simulink model "CTRL_ADAPT"  (R2023a)
settings: Solver=ode1  StartTime=0.0  StopTime=25  FixedStep=Ts  RelTol=1e-3
values from neighbouring files (symbols this model uses):
  Ts = 0.001    [TRAJ.m]
undefined symbols (not defined in the file or in its folder): DiscIntNeverNeededParam, PI0
settings Model: Creator=39388  LastModifiedBy=39388

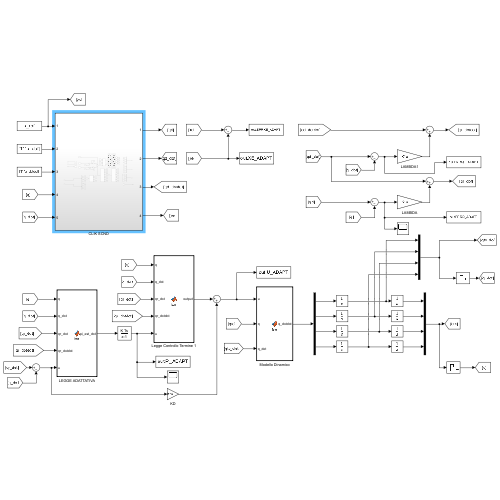
[thumbnail: Simulink's stored preview of the top-level diagram]
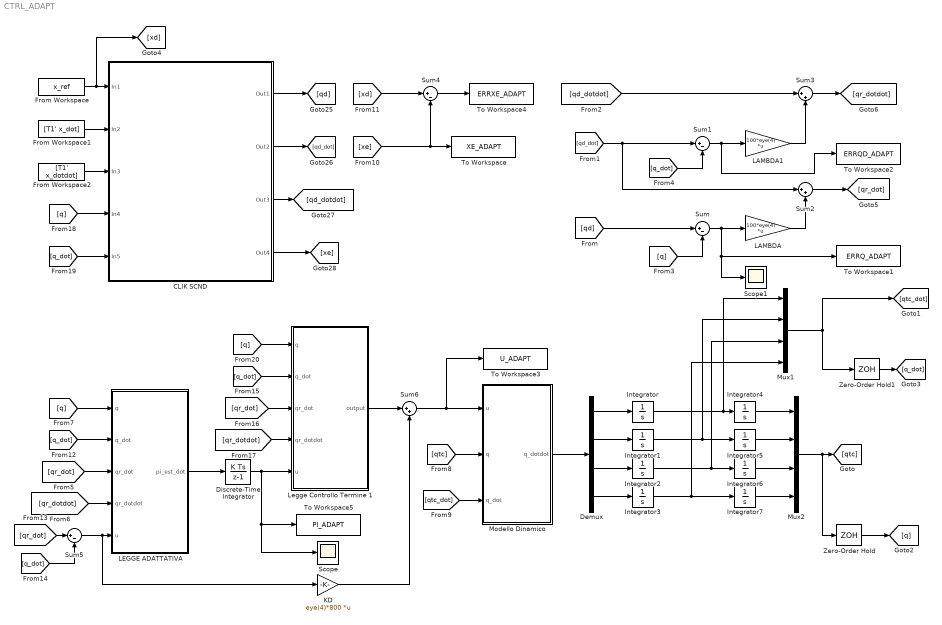
== system CTRL_ADAPT ==
  CLIK SCND : Subsystem
  Demux : Demux
  Discrete-Time Integrator : DiscreteIntegrator  InitialCondition=PI0'  SampleTime=Ts  ICPrevOutput=DiscIntNeverNeededParam  ICPrevScaledInput=DiscIntNeverNeededParam
  From Workspace : FromWorkspace  VariableName=x_ref  SampleTime=Ts
  From Workspace1 : FromWorkspace  VariableName=[T1' x_dot]  SampleTime=Ts
  From Workspace2 : FromWorkspace  VariableName=[T1' x_dotdot]  SampleTime=Ts
  Integrator : Integrator  UpperSaturationLimit=50  LowerSaturationLimit=-50
  Integrator{1..4} (4 alike) : Integrator
  Integrator5 : Integrator  InitialCondition=pi/2
  Integrator6 : Integrator  InitialCondition=-0.25
  Integrator7 : Integrator  InitialCondition=-pi
  KD : Gain  Gain=eye(4)*800  Multiplication=Matrix(K*u)
  LAMBDA : Gain  Gain=100*eye(4)  Multiplication=Matrix(K*u)
  LAMBDA1 : Gain  Gain=100*eye(4)  Multiplication=Matrix(K*u)
  LEGGE ADATTATIVA : MATLAB Function  TreatAsAtomicUnit=on
  Legge Controllo Termine 1 : MATLAB Function  TreatAsAtomicUnit=on
  Modello Dinamico : MATLAB Function  TreatAsAtomicUnit=on
  Mux1 : Mux
  Mux2 : Mux
  Scope : Scope
  Scope1 : Scope
  Sum{,1,4..5} (4 alike) : Sum  Inputs=|+-
  Sum2 : Sum  Inputs=|++
  Sum3 : Sum  Inputs=|++
  Sum6 : Sum  Inputs=|++
  To Workspace : ToWorkspace  VariableName=XE_ADAPT  SaveFormat=Structure With Time  SampleTime=-1
  To Workspace1 : ToWorkspace  VariableName=ERRQ_ADAPT  SaveFormat=Structure With Time  SampleTime=-1
  To Workspace2 : ToWorkspace  VariableName=ERRQD_ADAPT  SaveFormat=Structure With Time  SampleTime=-1
  To Workspace3 : ToWorkspace  VariableName=U_ADAPT  SaveFormat=Structure With Time  SampleTime=-1
  To Workspace4 : ToWorkspace  VariableName=ERRXE_ADAPT  SaveFormat=Structure With Time  SampleTime=-1
  To Workspace5 : ToWorkspace  VariableName=PI_ADAPT  SaveFormat=Structure With Time  SampleTime=-1
  Zero-Order Hold : ZeroOrderHold  SampleTime=Ts
  Zero-Order Hold1 : ZeroOrderHold  SampleTime=Ts
  wires:
  From Workspace/1 -> [xd], CLIK SCND/1(In1)
  From Workspace1/1 -> CLIK SCND/2(In2)
  From Workspace2/1 -> CLIK SCND/3(In3)
  [q] -> CLIK SCND/4(In4)
  [q_dot] -> CLIK SCND/5(In5)
  CLIK SCND/1(Out1) -> [qd]
  CLIK SCND/2(Out2) -> [qd_dot]
  CLIK SCND/3(Out3) -> [qd_dotdot]
  CLIK SCND/4(Out4) -> [xe]
  [qtc] -> Modello Dinamico/2(q)
  [qtc_dot] -> Modello Dinamico/3(q_dot)
  Modello Dinamico/1(q_dotdot) -> Demux/1
  Demux/1 -> Integrator/1
  Demux/2 -> Integrator1/1
  Demux/3 -> Integrator2/1
  Demux/4 -> Integrator3/1
  Integrator/1 -> Mux1/1, Integrator4/1
  Integrator1/1 -> Mux1/2, Integrator5/1
  Integrator2/1 -> Mux1/3, Integrator6/1
  Integrator3/1 -> Mux1/4, Integrator7/1
  Integrator4/1 -> Mux2/1
  Integrator5/1 -> Mux2/2
  Integrator6/1 -> Mux2/3
  Integrator7/1 -> Mux2/4
  Mux2/1 -> Zero-Order Hold/1, [qtc]
  Mux1/1 -> Zero-Order Hold1/1, [qtc_dot]
  Zero-Order Hold/1 -> [q]
  Zero-Order Hold1/1 -> [q_dot]
  [xe] -> Sum4/2, To Workspace/1
  [xd] -> Sum4/1
  Sum4/1 -> To Workspace4/1
  [qd_dot] -> Sum2/1, Sum1/1
  [q_dot] -> Sum1/2
  [qd] -> Sum/1
  [q] -> Sum/2
  Sum/1 -> Scope1/1, To Workspace1/1, LAMBDA/1
  LAMBDA/1 -> Sum2/2
  Sum2/1 -> [qr_dot]
  [qr_dot] -> LEGGE ADATTATIVA/3(qr_dot)
  Sum1/1 -> To Workspace2/1, LAMBDA1/1
  LAMBDA1/1 -> Sum3/2
  [qd_dotdot] -> Sum3/1
  Sum3/1 -> [qr_dotdot]
  [qr_dotdot] -> LEGGE ADATTATIVA/4(qr_dotdot)
  [q] -> LEGGE ADATTATIVA/1(q)
  [q_dot] -> LEGGE ADATTATIVA/2(q_dot)
  [q_dot] -> Sum5/2
  Sum5/1 -> KD/1, LEGGE ADATTATIVA/5(u)
  [qr_dot] -> Sum5/1
  LEGGE ADATTATIVA/1(pi_est_dot) -> Discrete-Time Integrator/1
  Discrete-Time Integrator/1 -> Scope/1, To Workspace5/1, Legge Controllo Termine 1/5(u)
  [q_dot] -> Legge Controllo Termine 1/2(q_dot)
  [qr_dot] -> Legge Controllo Termine 1/3(qr_dot)
  [q] -> Legge Controllo Termine 1/1(q)
  [qr_dotdot] -> Legge Controllo Termine 1/4(qr_dotdot)
  Sum6/1 -> To Workspace3/1, Modello Dinamico/1(u)
  Legge Controllo Termine 1/1(output) -> Sum6/1
  KD/1 -> Sum6/2

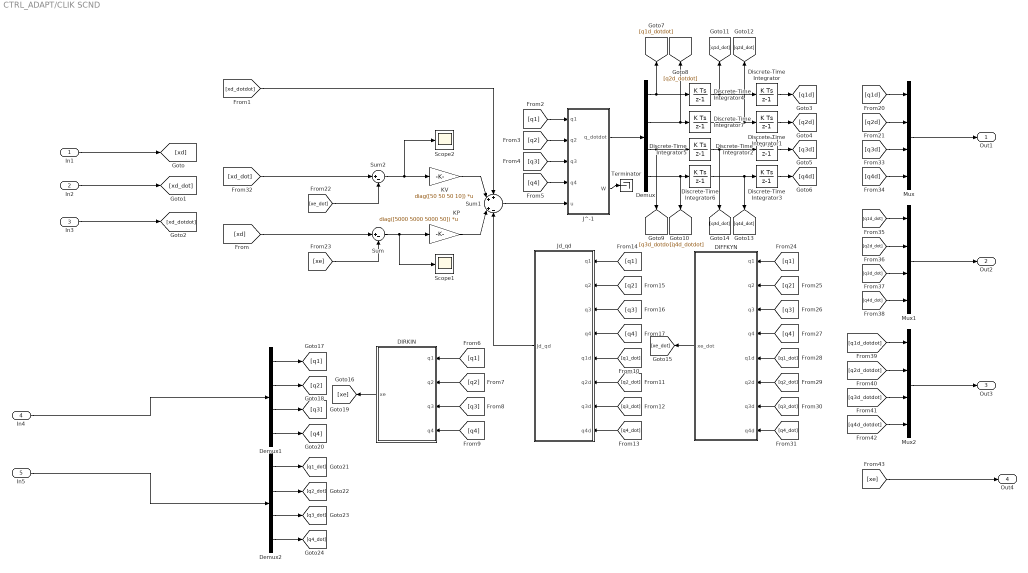
== system CTRL_ADAPT/CLIK SCND ==
  In1 : Inport
  In2 : Inport  Port=2
  In3 : Inport  Port=3
  In4 : Inport  Port=4
  In5 : Inport  Port=5
  DIFFKYN : MATLAB Function  TreatAsAtomicUnit=on
  DIRKIN : MATLAB Function  TreatAsAtomicUnit=on
  Demux : Demux
  Demux1 : Demux
  Demux2 : Demux
  Discrete-Time Integrator{,4..7} (5 alike) : DiscreteIntegrator  SampleTime=Ts  ICPrevOutput=DiscIntNeverNeededParam  ICPrevScaledInput=DiscIntNeverNeededParam
  Discrete-Time Integrator1 : DiscreteIntegrator  InitialCondition=pi/2  SampleTime=Ts  ICPrevOutput=DiscIntNeverNeededParam  ICPrevScaledInput=DiscIntNeverNeededParam
  Discrete-Time Integrator2 : DiscreteIntegrator  InitialCondition=-0.25  SampleTime=Ts  ICPrevOutput=DiscIntNeverNeededParam  ICPrevScaledInput=DiscIntNeverNeededParam
  Discrete-Time Integrator3 : DiscreteIntegrator  InitialCondition=-pi  SampleTime=Ts  ICPrevOutput=DiscIntNeverNeededParam  ICPrevScaledInput=DiscIntNeverNeededParam
  J^-1 : MATLAB Function  TreatAsAtomicUnit=on
  Jd_qd : MATLAB Function  TreatAsAtomicUnit=on
  KP : Gain  Gain=diag([5000 5000 5000 50])  Multiplication=Matrix(K*u)
  KV : Gain  Gain=diag([50 50 50 10])  Multiplication=Matrix(K*u)
  Mux : Mux
  Mux1 : Mux
  Mux2 : Mux
  Scope1 : Scope
  Scope2 : Scope
  Sum : Sum  Inputs=|+-
  Sum1 : Sum  Inputs=++|+-
  Sum2 : Sum  Inputs=|+-
  Terminator : Terminator
  Out1 : Outport
  Out2 : Outport  Port=2
  Out3 : Outport  Port=3
  Out4 : Outport  Port=4
  wires:
  [q4] -> J^-1/4(q4)
  [q1] -> DIFFKYN/1(q1)
  Demux/3 -> [q3d_dotdot], Discrete-Time Integrator5/1
  [q2d] -> Mux/2
  Discrete-Time Integrator1/1 -> [q2d]
  In5/1 -> Demux2/1
  [q1] -> DIRKIN/1(q1)
  [q4] -> DIRKIN/4(q4)
  Discrete-Time Integrator/1 -> [q1d]
  Demux/1 -> Discrete-Time Integrator4/1, [q1d_dotdot]
  Discrete-Time Integrator5/1 -> [q3d_dot], Discrete-Time Integrator2/1
  [xe_dot] -> Sum2/2
  [q3] -> J^-1/3(q3)
  [q3d] -> Mux/3
  Demux/4 -> [q4d_dotdot], Discrete-Time Integrator6/1
  [q1_dot] -> DIFFKYN/5(q1d)
  [q2] -> J^-1/2(q2)
  [q3] -> DIRKIN/3(q3)
  In2/1 -> [xd_dot]
  J^-1/1(q_dotdot) -> Demux/1
  Discrete-Time Integrator2/1 -> [q3d]
  [q2_dot] -> DIFFKYN/6(q2d)
  [xd] -> Sum/1
  Sum1/1 -> J^-1/5(u)
  [q4d] -> Mux/4
  KV/1 -> Sum1/2
  Jd_qd/1(Jd_qd) -> Sum1/4
  Discrete-Time Integrator3/1 -> [q4d]
  Discrete-Time Integrator4/1 -> [q1d_dot], Discrete-Time Integrator/1
  [q4d_dot] -> Mux1/4
  Demux1/3 -> [q3]
  Discrete-Time Integrator7/1 -> [q2d_dot], Discrete-Time Integrator1/1
  [xd_dotdot] -> Sum1/1
  [q2d_dot] -> Mux1/2
  Sum/1 -> Scope1/1, KP/1
  [xe] -> Sum/2
  Discrete-Time Integrator6/1 -> [q4d_dot], Discrete-Time Integrator3/1
  [q1] -> Jd_qd/1(q1)
  [q3_dot] -> DIFFKYN/7(q3d)
  [q2] -> DIFFKYN/2(q2)
  KP/1 -> Sum1/3
  [q3] -> Jd_qd/3(q3)
  In3/1 -> [xd_dotdot]
  [q3d_dot] -> Mux1/3
  DIRKIN/1(xe) -> [xe]
  [q3] -> DIFFKYN/3(q3)
  Demux1/2 -> [q2]
  [q1] -> J^-1/1(q1)
  [q2] -> Jd_qd/2(q2)
  Demux/2 -> [q2d_dotdot], Discrete-Time Integrator7/1
  [xe] -> Out4/1
  [q2] -> DIRKIN/2(q2)
  [q4_dot] -> DIFFKYN/8(q4d)
  [q4] -> Jd_qd/4(q4)
  DIFFKYN/1(xe_dot) -> [xe_dot]
  [xd_dot] -> Sum2/1
  J^-1/2(W) -> Terminator/1
  [q4] -> DIFFKYN/4(q4)
  Demux2/3 -> [q3_dot]
  Sum2/1 -> Scope2/1, KV/1
  [q3d_dotdot] -> Mux2/3
  [q1d_dot] -> Mux1/1
  [q1d] -> Mux/1
  Demux2/4 -> [q4_dot]
  Demux2/1 -> [q1_dot]
  Demux2/2 -> [q2_dot]
  [q4_dot] -> Jd_qd/8(q4d)
  [q1_dot] -> Jd_qd/5(q1d)
  [q3_dot] -> Jd_qd/7(q3d)
  [q2_dot] -> Jd_qd/6(q2d)
  [q1d_dotdot] -> Mux2/1
  [q4d_dotdot] -> Mux2/4
  [q2d_dotdot] -> Mux2/2
  Demux1/1 -> [q1]
  Demux1/4 -> [q4]
  In4/1 -> Demux1/1
  In1/1 -> [xd]
  Mux1/1 -> Out2/1
  Mux/1 -> Out1/1
  Mux2/1 -> Out3/1

== matlab function CTRL_ADAPT/CLIK SCND/DIRKIN ==
  data: q1 input; xe output; q2 input; q3 input; q4 input
function xe = fcn(q1,q2,q3,q4)

xe=[0.5*cos(q1)+0.5*cos(q1+q2);
    0.5*sin(q1)+0.5*sin(q1+q2);
    1+q3;
    q1+q2+q4];

== matlab function CTRL_ADAPT/CLIK SCND/J^-1 ==
  data: q1 input; q2 input; q3 input; q4 input; u input; q_dotdot output; W output
function  [q_dotdot,W] = fcn(q1,q2,q3,q4,u)

    J=[-0.5*sin(q1-0.5*sin(q1+q2)) -0.5*sin(q1+q2) 0 0;
        0.5*cos(q1-0.5*cos(q1+q2))  0.5*cos(q1+q2) 0 0;
        0                               0                 1 0;
        1                               1                 0 1];

     q_dotdot=J\u;
     
     W=0.5^2*abs(sin(q2));

== matlab function CTRL_ADAPT/CLIK SCND/Jd_qd ==
  data: q1 input; Jd_qd output; q2 input; q3 input; q4 input; q1d input; q2d input; q3d input; q4d input
function Jd_qd = fcn(q1,q2,q3,q4,q1d,q2d,q3d,q4d)

J_dot=[-0.5*q1d*cos(q1)-0.5*(q1d+q2d)*cos(q1+q2) -0.5*(q1d+q2d)*cos(q1+q2) 0 0;
       -0.5*q1d*sin(q1)-0.5*(q1d+q2d)*sin(q1+q2) -0.5*(q1d+q2d)*sin(q1+q2) 0 0;
        0                                         0                        0 0;
        0                                         0                        0 0];

Jd_qd=J_dot*[q1d; q2d; q3d; q4d];

== matlab function CTRL_ADAPT/CLIK SCND/DIFFKYN ==
  data: q1 input; xe_dot output; q2 input; q3 input; q4 input; q1d input; q2d input; q3d input; q4d input
function xe_dot = fcn(q1,q2,q3,q4,q1d,q2d,q3d,q4d)

J=[-0.5*sin(q1-0.5*sin(q1+q2)) -0.5*sin(q1+q2) 0 0;
    0.5*cos(q1-0.5*cos(q1+q2))  0.5*cos(q1+q2) 0 0;
    0                           0              1 0;
    1                           1              0 1];

xe_dot=J*[q1d;q2d;q3d;q4d];

== matlab function CTRL_ADAPT/LEGGE ADATTATIVA ==
  data: q input; pi_est_dot output; q_dot input; qr_dot input; qr_dotdot input; u input
function pi_est_dot = fcn(q,q_dot,qr_dot,qr_dotdot,u)

Kpi=eye(17)*100;
Kpi(6,6)=0.01;

q1=q(1);
q2=q(2);
q3=q(3);
q4=q(4);
qd1=q_dot(1);
qd2=q_dot(2);
qd3=q_dot(3);
qd4=q_dot(4);
qrd1=qr_dot(1);
qrd2=qr_dot(2);
qrd3=qr_dot(3);
qrd4=qr_dot(4);
qrdd1=qr_dotdot(1);
qrdd2=qr_dotdot(2);
qrdd3=qr_dotdot(3);
qrdd4=qr_dotdot(4);

Y=[(qrdd1*(2*cos(conj(q1))*cos(q1) + 2*sin(conj(q1))*sin(q1)))/2, qrdd1*((cos(conj(q1))*cos(q1))/4 + (sin(conj(q1))*sin(q1))/4), qrdd1*((cos(conj(q1))*cos(q1 + q2))/2 + (sin(conj(q1))*sin(q1 + q2))/2 + (cos(conj(q1) + conj(q2))*cos(q1))/2 + (sin(conj(q1) + conj(q2))*sin(q1))/2) + qrdd2*((cos(conj(q1))*cos(q1 + q2))/2 + (sin(conj(q1))*sin(q1 + q2))/2) - (qd2*qrd1*sin(q2))/2 - (qrd2*sin(q2)*(qd1 + qd2))/2, (qrdd1*(2*cos(conj(q1) + conj(q2))*cos(q1 + q2) + 2*sin(conj(q1) + conj(q2))*sin(q1 + q2)))/2 + (qrdd2*(2*cos(conj(q1) + conj(q2))*cos(q1 + q2) + 2*sin(conj(q1) + conj(q2))*sin(q1 + q2)))/2, qrdd1*((cos(q1 + q2)/2 + cos(q1)/2)*(cos(conj(q1))/2 + cos(conj(q1) + conj(q2))/2) + (sin(q1 + q2)/2 + sin(q1)/2)*(sin(conj(q1))/2 + sin(conj(q1) + conj(q2))/2)) + qrdd2*((cos(q1 + q2)*(cos(conj(q1))/2 + cos(conj(q1) + conj(q2))/2))/2 + (sin(q1 + q2)*(sin(conj(q1))/2 + sin(conj(q1) + conj(q2))/2))/2) - (qd2*qrd1*sin(q2))/4 - (qrd2*sin(q2)*(qd1 + qd2))/4, qrdd1*((cos(q1 + q2)/2 + cos(q1)/2)*(cos(conj(q1))/2 + cos(conj(q1) + conj(q2))/2) + (sin(q1 + q2)/2 + sin(q1)/2)*(sin(conj(q1))/2 + sin(conj(q1) + conj(q2))/2)) + qrdd2*((cos(q1 + q2)*(cos(conj(q1))/2 + cos(conj(q1) + conj(q2))/2))/2 + (sin(q1 + q2)*(sin(conj(q1))/2 + sin(conj(q1) + conj(q2))/2))/2) - (qd2*qrd1*sin(q2))/4 - (qrd2*sin(q2)*(qd1 + qd2))/4, qrdd1, qrdd1 + qrdd2, qrdd1 + qrdd2 + qrdd4, qrdd1, qrdd1 + qrdd2,         qrdd1 + qrdd2 + 50*qrdd3,        qrdd1 + qrdd2 + 20*qrdd4, qrd1,    0,         0,        0;
                                                            0,                                                             0,                                                                                                                                                                            qrdd1*((cos(conj(q1) + conj(q2))*cos(q1))/2 + (sin(conj(q1) + conj(q2))*sin(q1))/2) + (qd1*qrd1*sin(q2))/2, (qrdd1*(2*cos(conj(q1) + conj(q2))*cos(q1 + q2) + 2*sin(conj(q1) + conj(q2))*sin(q1 + q2)))/2 + (qrdd2*(2*cos(conj(q1) + conj(q2))*cos(q1 + q2) + 2*sin(conj(q1) + conj(q2))*sin(q1 + q2)))/2,                                                                                                                qrdd1*((cos(conj(q1) + conj(q2))*(cos(q1 + q2)/2 + cos(q1)/2))/2 + (sin(conj(q1) + conj(q2))*(sin(q1 + q2)/2 + sin(q1)/2))/2) + qrdd2*((cos(conj(q1) + conj(q2))*cos(q1 + q2))/4 + (sin(conj(q1) + conj(q2))*sin(q1 + q2))/4) + (qd1*qrd1*sin(q2))/4,                                                                                                                qrdd1*((cos(conj(q1) + conj(q2))*(cos(q1 + q2)/2 + cos(q1)/2))/2 + (sin(conj(q1) + conj(q2))*(sin(q1 + q2)/2 + sin(q1)/2))/2) + qrdd2*((cos(conj(q1) + conj(q2))*cos(q1 + q2))/4 + (sin(conj(q1) + conj(q2))*sin(q1 + q2))/4) + (qd1*qrd1*sin(q2))/4,     0, qrdd1 + qrdd2, qrdd1 + qrdd2 + qrdd4,     0, qrdd1 + qrdd2,         qrdd1 + qrdd2 + 50*qrdd3,        qrdd1 + qrdd2 + 20*qrdd4,    0, qrd2,         0,        0;
                                                            0,                                                             0,                                                                                                                                                                                                                                                                                     0,                                                                                                                                                                                             0,                                                                                                                                                                                                                                                                                                                                                     qrdd3 + 981/100,                                                                                                                                                                                                                                                                                                                                                     qrdd3 + 981/100,     0,             0,                     0,     0,             0, 50*qrdd1 + 50*qrdd2 + 2500*qrdd3,                               0,    0,    0, 2500*qrd3,        0;
                                                            0,                                                             0,                                                                                                                                                                                                                                                                                     0,                                                                                                                                                                                             0,                                                                                                                                                                                                                                                                                                                                                                   0,                                                                                                                                                                                                                                                                                                                                                                   0,     0,             0, qrdd1 + qrdd2 + qrdd4,     0,             0,                                0, 20*qrdd1 + 20*qrdd2 + 400*qrdd4,    0,    0,         0, 400*qrd4];
 
pi_est_dot = inv(Kpi)*Y'*u;

== matlab function CTRL_ADAPT/Legge Controllo Termine 1 ==
  data: q input size=4; output output size=4; q_dot input size=4; qr_dot input size=4; qr_dotdot input size=4; u input size=17
function output = fcn(q,q_dot,qr_dot,qr_dotdot,u)

q1=q(1);
q2=q(2);
q3=q(3);
q4=q(4);
qd1=q_dot(1);
qd2=q_dot(2);
qd3=q_dot(3);
qd4=q_dot(4);
qrd1=qr_dot(1);
qrd2=qr_dot(2);
qrd3=qr_dot(3);
qrd4=qr_dot(4);
qrdd1=qr_dotdot(1);
qrdd2=qr_dotdot(2);
qrdd3=qr_dotdot(3);
qrdd4=qr_dotdot(4);

Y=[(qrdd1*(2*cos(conj(q1))*cos(q1) + 2*sin(conj(q1))*sin(q1)))/2, qrdd1*((cos(conj(q1))*cos(q1))/4 + (sin(conj(q1))*sin(q1))/4), qrdd1*((cos(conj(q1))*cos(q1 + q2))/2 + (sin(conj(q1))*sin(q1 + q2))/2 + (cos(conj(q1) + conj(q2))*cos(q1))/2 + (sin(conj(q1) + conj(q2))*sin(q1))/2) + qrdd2*((cos(conj(q1))*cos(q1 + q2))/2 + (sin(conj(q1))*sin(q1 + q2))/2) - (qd2*qrd1*sin(q2))/2 - (qrd2*sin(q2)*(qd1 + qd2))/2, (qrdd1*(2*cos(conj(q1) + conj(q2))*cos(q1 + q2) + 2*sin(conj(q1) + conj(q2))*sin(q1 + q2)))/2 + (qrdd2*(2*cos(conj(q1) + conj(q2))*cos(q1 + q2) + 2*sin(conj(q1) + conj(q2))*sin(q1 + q2)))/2, qrdd1*((cos(q1 + q2)/2 + cos(q1)/2)*(cos(conj(q1))/2 + cos(conj(q1) + conj(q2))/2) + (sin(q1 + q2)/2 + sin(q1)/2)*(sin(conj(q1))/2 + sin(conj(q1) + conj(q2))/2)) + qrdd2*((cos(q1 + q2)*(cos(conj(q1))/2 + cos(conj(q1) + conj(q2))/2))/2 + (sin(q1 + q2)*(sin(conj(q1))/2 + sin(conj(q1) + conj(q2))/2))/2) - (qd2*qrd1*sin(q2))/4 - (qrd2*sin(q2)*(qd1 + qd2))/4, qrdd1*((cos(q1 + q2)/2 + cos(q1)/2)*(cos(conj(q1))/2 + cos(conj(q1) + conj(q2))/2) + (sin(q1 + q2)/2 + sin(q1)/2)*(sin(conj(q1))/2 + sin(conj(q1) + conj(q2))/2)) + qrdd2*((cos(q1 + q2)*(cos(conj(q1))/2 + cos(conj(q1) + conj(q2))/2))/2 + (sin(q1 + q2)*(sin(conj(q1))/2 + sin(conj(q1) + conj(q2))/2))/2) - (qd2*qrd1*sin(q2))/4 - (qrd2*sin(q2)*(qd1 + qd2))/4, qrdd1, qrdd1 + qrdd2, qrdd1 + qrdd2 + qrdd4, qrdd1, qrdd1 + qrdd2,         qrdd1 + qrdd2 + 50*qrdd3,        qrdd1 + qrdd2 + 20*qrdd4, qrd1,    0,         0,        0;
                                                            0,                                                             0,                                                                                                                                                                            qrdd1*((cos(conj(q1) + conj(q2))*cos(q1))/2 + (sin(conj(q1) + conj(q2))*sin(q1))/2) + (qd1*qrd1*sin(q2))/2, (qrdd1*(2*cos(conj(q1) + conj(q2))*cos(q1 + q2) + 2*sin(conj(q1) + conj(q2))*sin(q1 + q2)))/2 + (qrdd2*(2*cos(conj(q1) + conj(q2))*cos(q1 + q2) + 2*sin(conj(q1) + conj(q2))*sin(q1 + q2)))/2,                                                                                                                qrdd1*((cos(conj(q1) + conj(q2))*(cos(q1 + q2)/2 + cos(q1)/2))/2 + (sin(conj(q1) + conj(q2))*(sin(q1 + q2)/2 + sin(q1)/2))/2) + qrdd2*((cos(conj(q1) + conj(q2))*cos(q1 + q2))/4 + (sin(conj(q1) + conj(q2))*sin(q1 + q2))/4) + (qd1*qrd1*sin(q2))/4,                                                                                                                qrdd1*((cos(conj(q1) + conj(q2))*(cos(q1 + q2)/2 + cos(q1)/2))/2 + (sin(conj(q1) + conj(q2))*(sin(q1 + q2)/2 + sin(q1)/2))/2) + qrdd2*((cos(conj(q1) + conj(q2))*cos(q1 + q2))/4 + (sin(conj(q1) + conj(q2))*sin(q1 + q2))/4) + (qd1*qrd1*sin(q2))/4,     0, qrdd1 + qrdd2, qrdd1 + qrdd2 + qrdd4,     0, qrdd1 + qrdd2,         qrdd1 + qrdd2 + 50*qrdd3,        qrdd1 + qrdd2 + 20*qrdd4,    0, qrd2,         0,        0;
                                                            0,                                                             0,                                                                                                                                                                                                                                                                                     0,                                                                                                                                                                                             0,                                                                                                                                                                                                                                                                                                                                                     qrdd3 + 981/100,                                                                                                                                                                                                                                                                                                                                                     qrdd3 + 981/100,     0,             0,                     0,     0,             0, 50*qrdd1 + 50*qrdd2 + 2500*qrdd3,                               0,    0,    0, 2500*qrd3,        0;
                                                            0,                                                             0,                                                                                                                                                                                                                                                                                     0,                                                                                                                                                                                             0,                                                                                                                                                                                                                                                                                                                                                                   0,                                                                                                                                                                                                                                                                                                                                                                   0,     0,             0, qrdd1 + qrdd2 + qrdd4,     0,             0,                                0, 20*qrdd1 + 20*qrdd2 + 400*qrdd4,    0,    0,         0, 400*qrd4];
 
output = Y*u;

== matlab function CTRL_ADAPT/Modello Dinamico ==
  data: u input size=4; q_dotdot output size=4; q input size=4; q_dot input size=4
function q_dotdot= fcn(u,q,q_dot)

q1 = q(1);
q2 = q(2);
q3 = q(3);
q4 = q(4);
qd1 = q_dot(1);
qd2 = q_dot(2);
qd3 = q_dot(3);
qd4 = q_dot(4);

a1 = 0.5;
a2 = 0.5;
d0 = 1;

ml1 = 20;
ml2 = 20;
ml3 = 10;
m_load = 4;
Il1 = 4;
Il2 = 4;
Il4 = 1;
Im1 = 0.01;
Im2 = 0.01;
Im3 = 0.005;
Im4 = 0.001;
l1 = 0.25;
l2 = 0.25;
kr1 = 1;
kr2 = 1;
kr3 = 50;
kr4 = 20;
Fm1 =  0.00005;
Fm2 =  0.00005;
Fm3 = 0.01;
Fm4 = 0.005;

%% calcolo vettori posizione e assi z
p0 = [0 ; 0 ; d0];
p1 = [a1*cos(q1) ; a1*sin(q1) ; d0];
p2 = [a1*cos(q1) + a2*cos(q1+q2) ; a1*sin(q1) + a2*sin(q1+q2) ; d0];
p3 = p2 + [0 ; 0 ; q3]; % C'era un meno
p4 = p3;
pl1 = [l1*cos(q1) ; l1*sin(q1) ; d0];
pl2 = [a1*cos(q1) + l2*cos(q1+q2) ; a1*sin(q1) + l2*sin(q1+q2) ; d0];
pl3 = p3; 
pl4 = p4; 
z0 = [0 0 1]';
z1 = [0 0 1]';
z2 = [0 0 1]';
z3 = [0 0 1]';
z4 = [0 0 1]';

%% calcolo Jacobiani
Jp_l1 = [cross(z0,pl1-p0) zeros(3,3)];
Jp_l2 = [cross(z0,pl2-p0) cross(z1,pl2-p1) zeros(3,2)];
Jp_l3 = [cross(z0,pl3-p0) cross(z1,pl3-p1) z2 zeros(3,1)]; 
Jp_l4 = [cross(z0,pl4-p0) cross(z1,pl4-p1) z2 cross(z3,pl4-p3)]; %m4=mload

Jo_l1 = [z0 zeros(3,3)];
Jo_l2 = [z0 z1 zeros(3,2)];
Jo_l3 = [z0 z1 zeros(3,2)]; %Il3=0
Jo_l4 = [z0 z1 zeros(3,1) z3];


% Le masse dei motori sono trascurati, dunque ci concentriamo sulle parti
% angolari degli jacobiani.

Jo_m1 = Jo_l1;
Jo_m1(:,1) = kr1*z0;
Jo_m2 = Jo_l2;  
Jo_m2(:,2) = kr2*z1;
Jo_m3 = Jo_l3; 
Jo_m3(:,3) = kr3*z2;
Jo_m4 = Jo_l4;  
Jo_m4(:,4) = kr4*z3;


%% calcolo B

B1 = ml1*(Jp_l1'*Jp_l1) + Il1*(Jo_l1'*Jo_l1) + Im1*(Jo_m1'*Jo_m1); 
B2 = ml2*(Jp_l2'*Jp_l2) + Il2*(Jo_l2'*Jo_l2) + Im2*(Jo_m2'*Jo_m2); 
B3 = ml3*(Jp_l3'*Jp_l3) + 0 + Im3*(Jo_m3'*Jo_m3); %Il3=0
B4 = m_load*(Jp_l4'*Jp_l4) + Il4*(Jo_l4'*Jo_l4) + Im4*(Jo_m4'*Jo_m4); 

B = B1 + B2 + B3 + B4;

%% calcolo C

C = [-a1*qd2*sin(q2)*(a2*m_load + a2*ml3 + l2*ml2), -a1*sin(q2)*(qd1 + qd2)*(a2*m_load + a2*ml3 + l2*ml2), 0, 0;
      a1*qd1*sin(q2)*(a2*m_load + a2*ml3 + l2*ml2),  0, 0, 0;
      0, 0, 0, 0;
      0, 0, 0, 0]; 

%% calcolo Fv

Fv = diag([kr1^2*Fm1 kr2^2*Fm2 kr3^2*Fm3 kr4^2*Fm4]);

%% calcolo g

g0 = [0 0 -9.81]';
g1 = - (ml1*g0'*Jp_l1(:,1) + ml2*g0'*Jp_l2(:,1) + ml3*g0'*Jp_l3(:,1) + m_load*g0'*Jp_l4(:,1));
g2 = - (ml1*g0'*Jp_l1(:,2) + ml2*g0'*Jp_l2(:,2) + ml3*g0'*Jp_l3(:,2) + m_load*g0'*Jp_l4(:,2));
g3 = - (ml1*g0'*Jp_l1(:,3) + ml2*g0'*Jp_l2(:,3) + ml3*g0'*Jp_l3(:,3) + m_load*g0'*Jp_l4(:,3));
g4 = - (ml1*g0'*Jp_l1(:,4) + ml2*g0'*Jp_l2(:,4) + ml3*g0'*Jp_l3(:,4) + m_load*g0'*Jp_l4(:,4));
g = [g1 g2 g3 g4]';

%% Risultato

q_d=[qd1; qd2; qd3; qd4];

q_dotdot=inv(B)*(u-C*q_d-Fv*q_d-g);
